simulink model "bpsk6"  (R2021b)
settings: Solver=VariableStepAuto  StartTime=0.0  StopTime=500  RelTol=1e-3
libraries: dsp_blocks x5
settings Model: Creator=aidynardabek  LastModifiedBy=aidynardabek

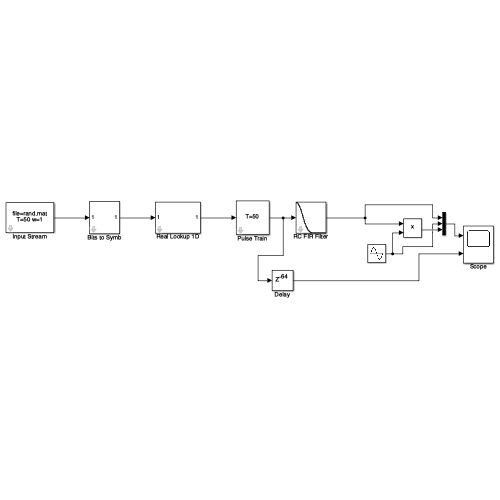
[thumbnail: Simulink's stored preview of the top-level diagram]
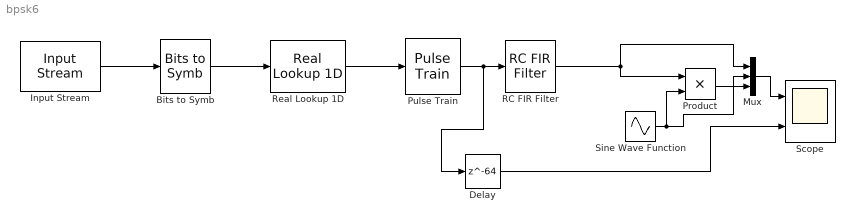
== system bpsk6 ==
  Bits to Symb : dsp_blocks/Conversions/Bits to Symb
  Delay : Delay  DelayLength=64
  Input Stream : dsp_blocks/Sources//Sinks/Input Stream  period=50  width=1  fname=rand.mat
  Mux : Mux  Inputs=3
  Product : Product
  Pulse Train : dsp_blocks/Conversions/Pulse Train  period=50
  RC FIR Filter : dsp_blocks/Filters/RC FIR Filter  period=50  beta=0.5  root=off  filt_len=128  win_type=on
  Real Lookup 1D : dsp_blocks/Conversions/Real Lookup 1D  table=[-1 1]
  Scope : Scope  NumInputPorts=2
  Sine Wave Function : Sin  Frequency=2*pi*0.1  SampleTime=0
  wires:
  Bits to Symb/1 -> Real Lookup 1D/1
  Input Stream/1 -> Bits to Symb/1
  Pulse Train/1 -> Delay/1, RC FIR Filter/1
  Real Lookup 1D/1 -> Pulse Train/1
  Delay/1 -> Scope/2
  Mux/1 -> Scope/1
  Product/1 -> Mux/3
  Sine Wave Function/1 -> Product/2, Mux/2
  RC FIR Filter/1 -> Mux/1, Product/1
